simulink model "Simulation"  (R2026a)
settings: Solver=VariableStepAuto
libraries: simulink x1, simulink_extras x1, shared3dof x1
settings Model: Creator=jdharc  LastModifiedBy=jdharc

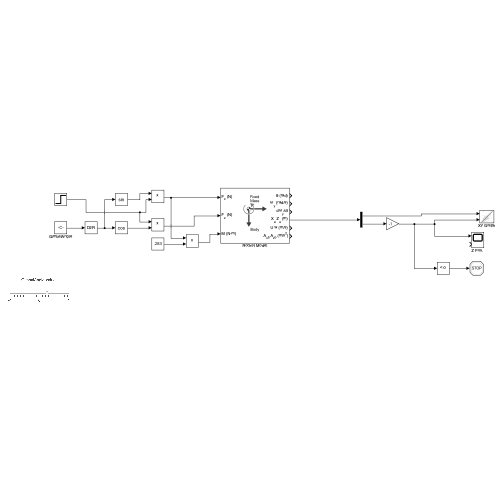
[thumbnail: Simulink's stored preview of the top-level diagram]
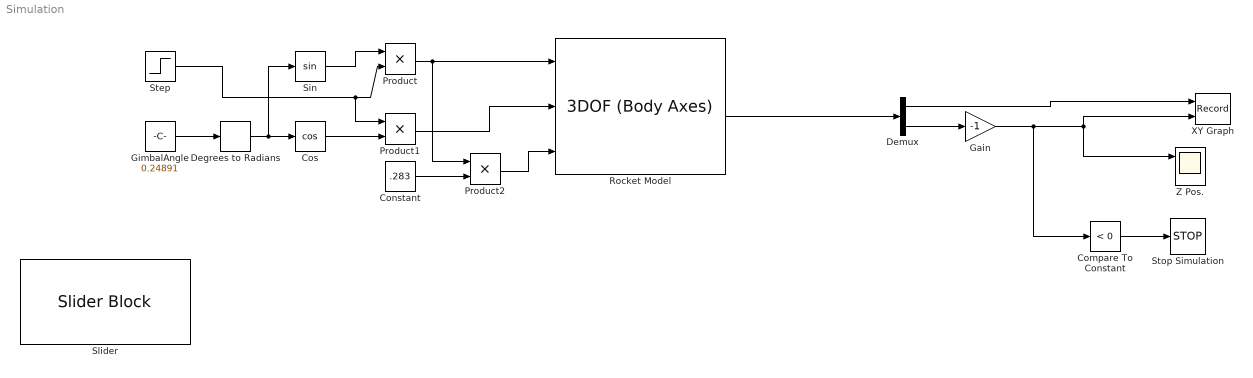
== system Simulation ==
  Compare To Constant : simulink/Logic and Bit Operations/Compare To Constant  relop=<  const=0  OutDataTypeStr=boolean
  Constant : Constant  Value=.283
  Cos : Trigonometry  Operator=cos
  Degrees to Radians : simulink_extras/Transformations/Degrees to Radians
  Demux : Demux  Outputs=2
  Gain : Gain  Gain=-1
  GimbalAngle : Constant  Value=0.24891
  Product : Product
  Product1 : Product
  Product2 : Product
  Rocket Model : shared3dof/3DOF (Body Axes)  units=Metric (MKS)  mtype=Fixed  v_ini=0  theta_ini=0  alpha_ini=0  pos_ini=[0 0]  q_ini=0  mass=.892  mass_e=0.5  mass_f=3.0  Iyy=0.286  Iyy_e=0.5  Iyy_f=3.0  g_in=Internal  g=9.81  vre_flag=on  abi_flag=off  aMode=0  vel_statename=''  theta_statename=''  pos_statename=''  q_statename=''  mass_statename=''
  Sin : Trigonometry
  Slider : SliderBlock  ScaleMin=-1  ScaleMax=1  TickInterval=1
  Step : Step  SampleTime=0
  Stop Simulation : Stop
  XY Graph : Record  NumPorts=2.0  FileSettingsInternal="{\"entries\":[{\"content\":{\"excelSettings\":{\"content\":{},\"type\":\"Streamout.ExcelSettings\"},\"parquetSettings\":{\"content\":{},\"type\":\"Streamout.ParquetSettings\"}},\"type\":\"Streamout.FileSettingStorage\",\"uuid\":\"\"}],\"packageUris\":[\"http:\\/\\/schema.mathworks.com\\/mf0\\/streamout_blocks\\/R2020a\"],\"version\":\"1.0\"}"  FrameSettings=[0, 0]  Layout=[1 1]  SignalsInternal="{\"entries\":[{\"content\":{\"signals\":[{\"content\":{\"blockPath\":[],\"dimensions\":[1],\"domain\":\"\",\"lineColor\":\"#64d413\",\"lineWidth\":2,\"port\":1,\"sid\":[\"\"],\"signalID\":1,\"signalName\":\"Demux:1\"},\"type\":\"RecordBlkView.Signal\",\"uuid\":\"\"},{\"content\":{\"blockPath\":[],\"dimensions\":[1],\"domain\":\"\",\"lineColor\":\"#ff13a6\",\"lineWidth\":2,\"port\":2,\"sid\":[\"\"],\"signalID\":2,\"signalName\":\"Gain\"},\"type\":\"RecordBlkView.Signal\",\"uuid\":\"\"}]},\"type\":\"RecordBlkView.InputSignals\",\"uuid\":\"\"}],\"packageUris\":[\"http:\\/\\/schema.mathworks.com\\/mf0\\/streamout_blocks\\/R2020a\"],\"version\":\"1.0\"}"  VisualizationBindings="{\"xyplotplugin\":{\"info\":[{\"series\":[],\"subplotID\":1}]}}"  CompatibilityTag=XY
  Z Pos. : Scope  NumInputPorts=2
      settings: ActiveDisplayYMinimum=32.0746661299055  ActiveDisplayYMaximum=181.90961038047436
  wires:
  Rocket Model/4 -> Demux/1
  Demux/2 -> Gain/1
  Demux/1 -> XY Graph/1
  Gain/1 -> Compare To Constant/1, XY Graph/2, Z Pos./1
  Compare To Constant/1 -> Stop Simulation/1
  GimbalAngle/1 -> Degrees to Radians/1
  Degrees to Radians/1 -> Sin/1, Cos/1
  Sin/1 -> Product/1
  Cos/1 -> Product1/2
  Step/1 -> Product1/1, Product/2
  Product/1 -> Product2/1, Rocket Model/1
  Product1/1 -> Rocket Model/2
  Constant/1 -> Product2/2
  Product2/1 -> Rocket Model/3
